simulink model "bldc_sim_abcFrame"  (R2024b)
settings: Solver=VariableStepAuto  StartTime=0.0  StopTime=2  RelTol=1e-3
values from neighbouring files (symbols this model uses):
  D_m = 1e-5    (= 1e-05)    [setup_motor_params.m]
  J = 12e-4    (= 0.0012)    [setup_motor_params.m]
  Ke = 0.1    [setup_motor_params.m]
  L_ss = 0.45e-3    (= 0.00045)    [setup_motor_params.m]
  P = 8    [setup_motor_params.m]
  phi_A_deg = 9.0 * 0    (= 0)    [setup_motor_params.m]
  phi_B_deg = -1.0 * 0    (= 0)    [setup_motor_params.m]
  phi_C_deg = 7.0* 0    (= 0)    [setup_motor_params.m]
  R_s = 0.15    [setup_motor_params.m]
  Ts_motor = 1e-6    (= 1e-06)    [setup_motor_params.m]
libraries: nesl_utility x12, ee_lib x6, fl_lib x5, embmathops x1, spsPWMGeneratorDCDCLib x1, simulink x1
settings Model: Creator=Aether  LastModifiedBy=Aether

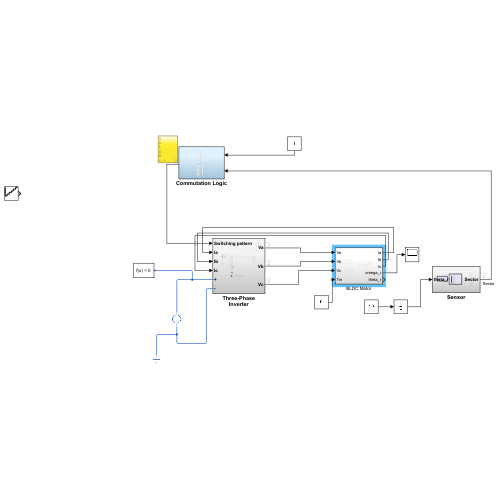
[thumbnail: Simulink's stored preview of the top-level diagram]
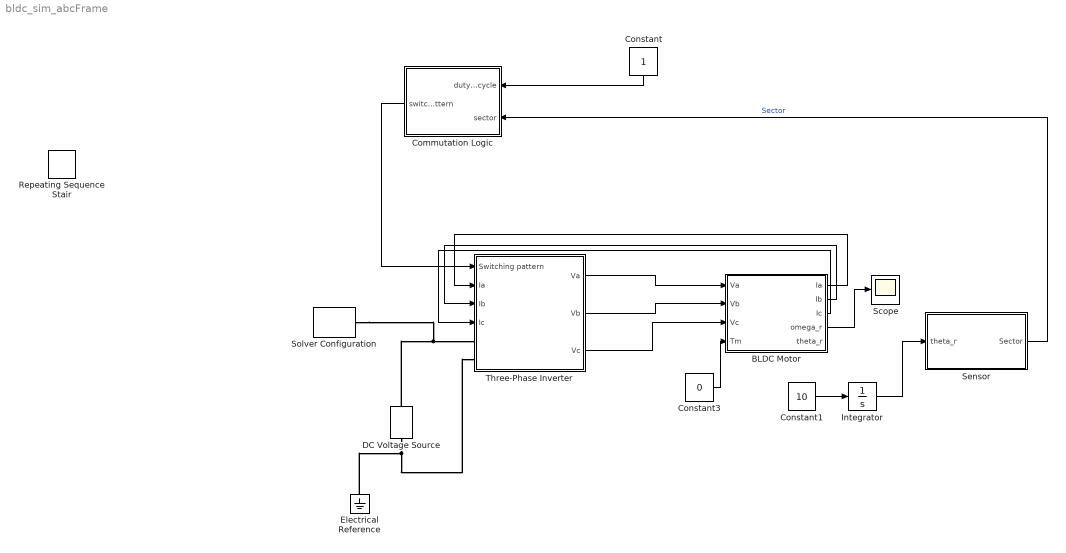
== system bldc_sim_abcFrame ==
  BLDC Motor : Subsystem
  Commutation Logic : Subsystem
  Constant : Constant
  Constant1 : Constant  Value=10
  Constant3 : Constant  Value=0
  DC Voltage Source : ee_lib/Additional Components/SPICE Sources/DC Voltage Source  DC=36 V
  Electrical Reference : fl_lib/Electrical/Electrical Elements/Electrical Reference
  Integrator : Integrator
  Repeating Sequence Stair : simulink/Sources/Repeating Sequence Stair  OutValues=[1 2 3 4 5 6]  tsamp=0.02  OutMin=[]  OutMax=[]  OutDataTypeStr=double  OutputDataTypeScalingMode=double  OutDataType=fixdt(0,8)  ConRadixGroup=Best Precision: Vector-wise  OutScaling=2^-12
  Scope : Scope
  Sensor : Subsystem
  Solver Configuration : nesl_utility/Solver Configuration  PhysicalDomain=network_engine_domain  SubClassName=solver  LeftPortType=input  RightPortType=generic  Tones=[]  Harmonics=[]  SimulateNoise=off  Profile=off  UseLocalSampling=off  EnableSwitchedLinearOptims=on  FrequencyDomain=off  UseCCode=off  RelTol=0.001  AbsTol=0.001  MinStep=1e-09  ToWorkspace=off  RevertToSquareIcSolve=off  NumHomotopyIterations=100  PhasorMode=off  PhasorModeNumHarmonics=1  ConsistencySolver=NEWTON_XTOL_AFTER_FTOL  IndexReductionMethod=DerivativeReplacement  DoDC=off  ResidualTolerance=1e-09  ConsistencyTolSource=GLOBAL  ConsistencyAbsTol=0.001  ConsistencyRelTol=0.001  ConsistencyTolFactor=0.001  UseLocalSolver=off  LocalSolverChoice=NE_BACKWARD_EULER_ADVANCER  ResolveIndetEquations=on  FunctionEvalNumThread=1  LocalSolverSampleTime=0.001  DoFixedCost=off  MaxNonlinIter=3  MaxModeIter=2  ComputeImpulses=off  ImpulseIterations=2  LinearAlgebra=auto  LinearAlgebraNumThread=0  EquationFormulation=NE_TIME_EF  DelaysMemoryBudget=1024  AutomaticFiltering=on  FilteringTimeConstant=0.001  PartitionStorageMethod=AS_NEEDED  PartitionMemoryBudget=1024  PartitionMethod=ROBUST  MultibodyUseLocalSolver=off  MultibodyLocalSolverChoice=ODE1  MultibodyLocalSolverSampleTime=0.001
  Three-Phase Inverter : Subsystem
  wires:
  Constant3/1 -> BLDC Motor/4(Tm)
  Constant/1 -> Commutation Logic/1(duty_cycle)
  BLDC Motor/1(Ia) -> Three-Phase Inverter/2(Ia)
  BLDC Motor/2(Ib) -> Three-Phase Inverter/3(Ib)
  BLDC Motor/3(Ic) -> Three-Phase Inverter/4(Ic)
  Three-Phase Inverter/1(Va) -> BLDC Motor/1(Va)
  Three-Phase Inverter/2(Vb) -> BLDC Motor/2(Vb)
  Three-Phase Inverter/3(Vc) -> BLDC Motor/3(Vc)
  BLDC Motor/4(omega_r) -> Scope/1
  Commutation Logic/1("  switching_pattern") -> Three-Phase Inverter/1(Switching pattern)
  Sensor/1(Sector) -> Commutation Logic/2(sector)  "Sector"
  Constant1/1 -> Integrator/1
  Integrator/1 -> Sensor/1(theta_r)
  connections:
  DC Voltage Source/LConn1 -- Solver Configuration/RConn1 -- Three-Phase Inverter/LConn1
  DC Voltage Source/RConn1 -- Electrical Reference/LConn1 -- Three-Phase Inverter/LConn2

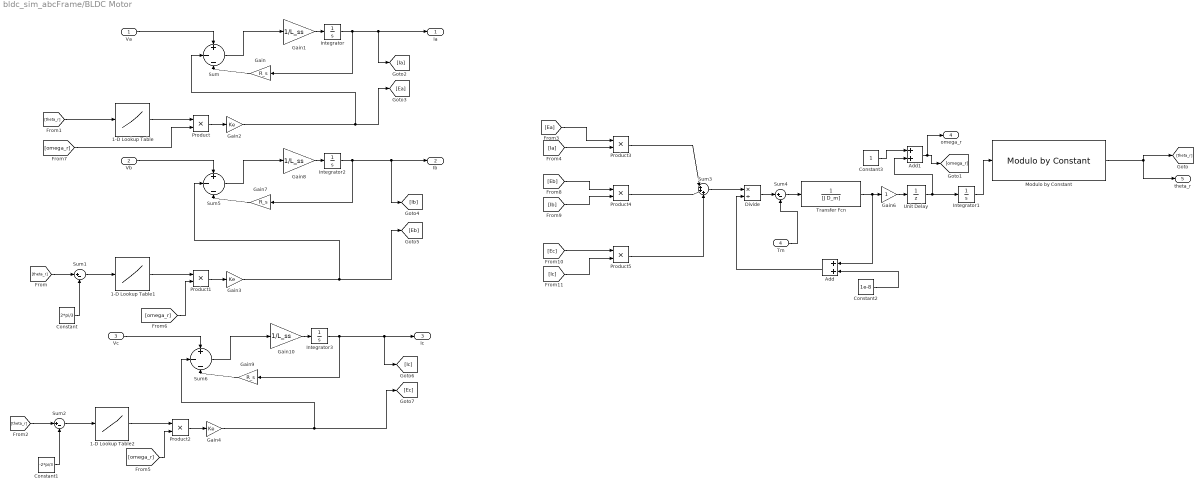
== system bldc_sim_abcFrame/BLDC Motor ==
  Va : Inport
  Vb : Inport  Port=2
  Vc : Inport  Port=3
  Tm : Inport  Port=4
  1-D Lookup Table : Lookup_n-D  NumberOfTableDimensions=1  BreakpointsForDimension1=[0, pi/3, 2*pi/3, pi, 4*pi/3, 5*pi/3, 2*pi]  Table=[0, 1, 1, 0, -1, -1, 0]  InternalRulePriority=Speed  RndMeth=Simplest
  1-D Lookup Table1 : Lookup_n-D  NumberOfTableDimensions=1  BreakpointsForDimension1=[0, pi/3, 2*pi/3, pi, 4*pi/3, 5*pi/3, 2*pi]  Table=[0, 1, 1, 0, -1, -1, 0]  InternalRulePriority=Speed  RndMeth=Simplest
  1-D Lookup Table2 : Lookup_n-D  NumberOfTableDimensions=1  BreakpointsForDimension1=[0, pi/3, 2*pi/3, pi, 4*pi/3, 5*pi/3, 2*pi]  Table=[0, 1, 1, 0, -1, -1, 0]  InternalRulePriority=Speed  RndMeth=Simplest
  Add : Sum
  Add1 : Sum
  Constant : Constant  Value=2*pi/3
  Constant1 : Constant  Value=-2*pi/3
  Constant2 : Constant  Value=1e-8
  Constant3 : Constant
  Divide : Product  Inputs=*/
  Gain : Gain  Gain=R_s
  Gain1 : Gain  Gain=1/L_ss
  Gain10 : Gain  Gain=1/L_ss
  Gain2 : Gain  Gain=Ke
  Gain3 : Gain  Gain=Ke
  Gain4 : Gain  Gain=Ke
  Gain6 : Gain
  Gain7 : Gain  Gain=R_s
  Gain8 : Gain  Gain=1/L_ss
  Gain9 : Gain  Gain=R_s
  Integrator : Integrator
  Integrator1 : Integrator  InitialCondition=0.1
  Integrator2 : Integrator
  Integrator3 : Integrator
  Modulo by Constant : embmathops/Modulo by Constant  Denominator=2*pi  SimulateUsing=Code generation
  Product{,1..5} (6 alike) : Product
  Sum : Sum  Inputs=+|-|-
  Sum1 : Sum  Inputs=|+-
  Sum2 : Sum  Inputs=|+-
  Sum3 : Sum  Inputs=|+++
  Sum4 : Sum  Inputs=|+-
  Sum5 : Sum  Inputs=+|-|-
  Sum6 : Sum  Inputs=+|-|-
  Transfer Fcn : TransferFcn  Denominator=[J D_m]
  Unit Delay : UnitDelay  SampleTime=-1  HasFrameUpgradeWarning=on
  Ia : Outport
  Ib : Outport  Port=2
  Ic : Outport  Port=3
  omega_r : Outport  Port=4
  theta_r : Outport  Port=5
  wires:
  Va/1 -> Sum/1
  Gain/1 -> Sum/3
  Sum/1 -> Gain1/1
  Gain1/1 -> Integrator/1
  Integrator/1 -> [Ia], Ia/1, Gain/1
  1-D Lookup Table/1 -> Product/1
  Product/1 -> Gain2/1
  Gain2/1 -> Sum/2, [Ea]
  Product1/1 -> Gain3/1
  1-D Lookup Table1/1 -> Product1/1
  Sum1/1 -> 1-D Lookup Table1/1
  Constant/1 -> Sum1/2
  Constant1/1 -> Sum2/2
  1-D Lookup Table2/1 -> Product2/1
  Product2/1 -> Gain4/1
  Sum2/1 -> 1-D Lookup Table2/1
  Product3/1 -> Sum3/1
  Product4/1 -> Sum3/2
  Product5/1 -> Sum3/3
  Sum3/1 -> Divide/1
  Divide/1 -> Sum4/1
  Tm/1 -> Sum4/2
  Sum4/1 -> Transfer Fcn/1
  Transfer Fcn/1 -> Gain6/1, Add/1
  Integrator1/1 -> Modulo by Constant/1
  Gain7/1 -> Sum5/3
  Gain8/1 -> Integrator2/1
  Sum5/1 -> Gain8/1
  Vb/1 -> Sum5/1
  Vc/1 -> Sum6/1
  Gain9/1 -> Sum6/3
  Gain10/1 -> Integrator3/1
  Sum6/1 -> Gain10/1
  Modulo by Constant/1 -> theta_r/1, [theta_r]
  [theta_r] -> Sum1/1
  [theta_r] -> Sum2/1
  [omega_r] -> Product2/2
  [omega_r] -> Product1/2
  [omega_r] -> Product/2
  [theta_r] -> 1-D Lookup Table/1
  Constant2/1 -> Add/2
  Add/1 -> Divide/2
  Gain3/1 -> Sum5/2, [Eb]
  Integrator2/1 -> [Ib], Ib/1, Gain7/1
  Integrator3/1 -> [Ic], Ic/1, Gain9/1
  Gain4/1 -> Sum6/2, [Ec]
  [Ea] -> Product3/1
  [Ia] -> Product3/2
  [Eb] -> Product4/1
  [Ib] -> Product4/2
  [Ec] -> Product5/1
  [Ic] -> Product5/2
  Gain6/1 -> Unit Delay/1
  Unit Delay/1 -> Integrator1/1, Add1/2
  Constant3/1 -> Add1/1
  Add1/1 -> omega_r/1, [omega_r]

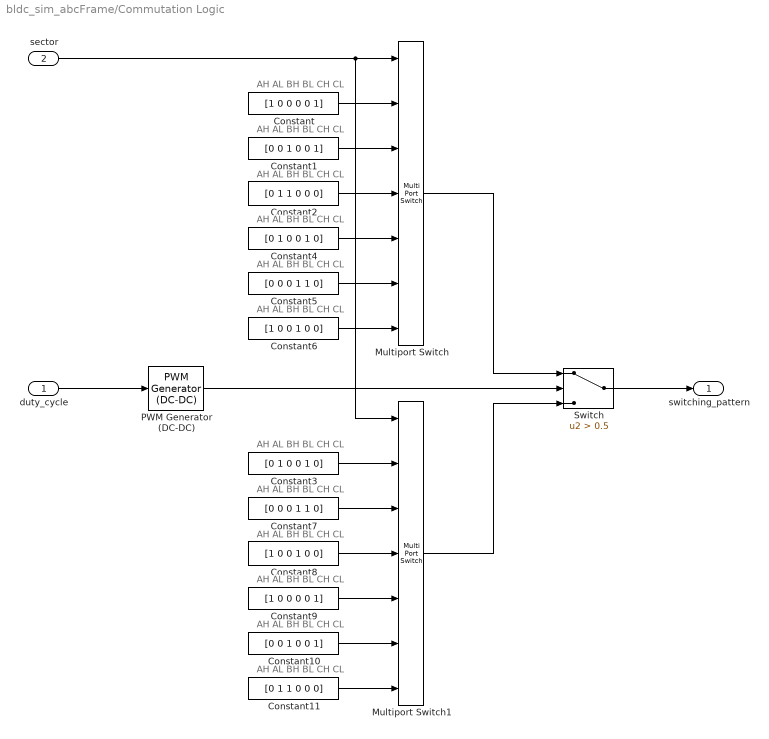
== system bldc_sim_abcFrame/Commutation Logic ==
  note: AH AL BH BL CH CL
  note: AH AL BH BL CH CL
  note: AH AL BH BL CH CL
  note: AH AL BH BL CH CL
  note: AH AL BH BL CH CL
  note: AH AL BH BL CH CL
  note: AH AL BH BL CH CL
  note: AH AL BH BL CH CL
  note: AH AL BH BL CH CL
  note: AH AL BH BL CH CL
  note: AH AL BH BL CH CL
  note: AH AL BH BL CH CL
  duty_cycle : Inport
  sector : Inport  Port=2
  Constant : Constant  Value=[1 0 0 0 0 1]
  Constant1 : Constant  Value=[0 0 1 0 0 1]
  Constant10 : Constant  Value=[0 0 1 0 0 1]
  Constant11 : Constant  Value=[0 1 1 0 0 0]
  Constant2 : Constant  Value=[0 1 1 0 0 0]
  Constant3 : Constant  Value=[0 1 0 0 1 0]
  Constant4 : Constant  Value=[0 1 0 0 1 0]
  Constant5 : Constant  Value=[0 0 0 1 1 0]
  Constant6 : Constant  Value=[1 0 0 1 0 0]
  Constant7 : Constant  Value=[0 0 0 1 1 0]
  Constant8 : Constant  Value=[1 0 0 1 0 0]
  Constant9 : Constant  Value=[1 0 0 0 0 1]
  Multiport Switch : MultiPortSwitch  Inputs=6  SaturateOnIntegerOverflow=off  InputSameDT=off
  Multiport Switch1 : MultiPortSwitch  Inputs=6  SaturateOnIntegerOverflow=off  InputSameDT=off
  PWM Generator (DC-DC) : spsPWMGeneratorDCDCLib/PWM Generator (DC-DC)  Fsw=1e7  Ts=Ts_motor
  Switch : Switch  Criteria=u2 > Threshold  Threshold=0.5  SaturateOnIntegerOverflow=off  InputSameDT=off
  "  switching_pattern" : Outport  VectorParamsAs1DForOutWhenUnconnected=off
  wires:
  Constant6/1 -> Multiport Switch/7
  Constant4/1 -> Multiport Switch/5
  sector/1 -> Multiport Switch1/1, Multiport Switch/1
  Constant1/1 -> Multiport Switch/3
  Constant2/1 -> Multiport Switch/4
  Constant5/1 -> Multiport Switch/6
  Constant/1 -> Multiport Switch/2
  Constant9/1 -> Multiport Switch1/5
  Constant11/1 -> Multiport Switch1/7
  Constant3/1 -> Multiport Switch1/2
  Constant7/1 -> Multiport Switch1/3
  Constant10/1 -> Multiport Switch1/6
  Constant8/1 -> Multiport Switch1/4
  PWM Generator (DC-DC)/1 -> Switch/2
  Switch/1 -> "  switching_pattern"/1
  Multiport Switch/1 -> Switch/1
  Multiport Switch1/1 -> Switch/3
  duty_cycle/1 -> PWM Generator (DC-DC)/1

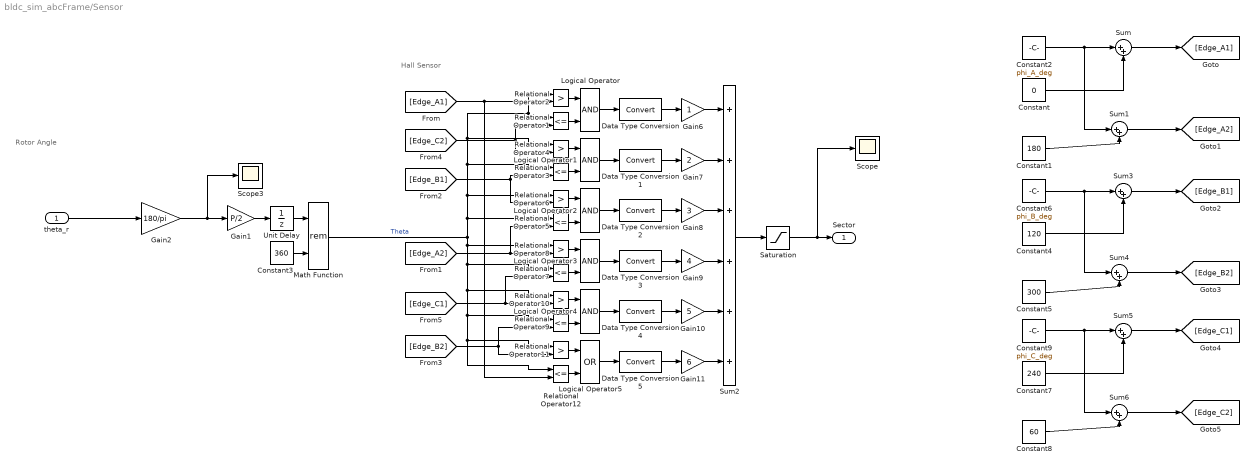
== system bldc_sim_abcFrame/Sensor ==
  note: Rotor Angle
  note: Hall Sensor
  theta_r : Inport
  Constant : Constant  Value=0
  Constant1 : Constant  Value=180
  Constant2 : Constant  Value=phi_A_deg
  Constant3 : Constant  Value=360
  Constant4 : Constant  Value=120
  Constant5 : Constant  Value=300
  Constant6 : Constant  Value=phi_B_deg
  Constant7 : Constant  Value=240
  Constant8 : Constant  Value=60
  Constant9 : Constant  Value=phi_C_deg
  Data Type Conversion{,1..5} (6 alike) : DataTypeConversion
  Gain1 : Gain  Gain=P/2
  Gain10 : Gain  Gain=5  SaturateOnIntegerOverflow=on  OutDataTypeStr=Inherit: Same as input  ParamDataTypeStr=Inherit: Same as input
  Gain11 : Gain  Gain=6  SaturateOnIntegerOverflow=on  OutDataTypeStr=Inherit: Same as input  ParamDataTypeStr=Inherit: Same as input
  Gain2 : Gain  Gain=180/pi
  Gain6 : Gain  SaturateOnIntegerOverflow=on  OutDataTypeStr=Inherit: Same as input  ParamDataTypeStr=Inherit: Same as input
  Gain7 : Gain  Gain=2  SaturateOnIntegerOverflow=on  OutDataTypeStr=Inherit: Same as input  ParamDataTypeStr=Inherit: Same as input
  Gain8 : Gain  Gain=3  SaturateOnIntegerOverflow=on  OutDataTypeStr=Inherit: Same as input  ParamDataTypeStr=Inherit: Same as input
  Gain9 : Gain  Gain=4  SaturateOnIntegerOverflow=on  OutDataTypeStr=Inherit: Same as input  ParamDataTypeStr=Inherit: Same as input
  Logical Operator{,1..4} (5 alike) : Logic
  Logical Operator5 : Logic  Operator=OR
  Math Function : Math  Operator=rem  SignedPower=on
  Relational Operator{1,3,5,7,9,12} (6 alike) : RelationalOperator  Operator=<=
  Relational Operator{2,4,6,8,10..11} (6 alike) : RelationalOperator  Operator=>
  Saturation : Saturate  UpperLimit=6  LowerLimit=1
  Scope : Scope
  Scope3 : Scope
  Sum{,1,3..6} (6 alike) : Sum  Inputs=|++
  Sum2 : Sum  Inputs=++++++  InputSameDT=on  SaturateOnIntegerOverflow=on  OutDataTypeStr=Inherit: Same as first input
  Unit Delay : UnitDelay  SampleTime=Ts_motor  HasFrameUpgradeWarning=on
  Sector : Outport
  wires:
  Saturation/1 -> Scope/1, Sector/1
  Math Function/1 -> Relational Operator2/1, Relational Operator1/1, Relational Operator4/1, Relational Operator3/1, Relational Operator6/1, Relational Operator5/1, Relational Operator12/1, Relational Operator11/1, Relational Operator9/1, Relational Operator10/1, Relational Operator7/1, Relational Operator8/1  "Theta"
  Data Type Conversion5/1 -> Gain11/1
  Data Type Conversion4/1 -> Gain10/1
  Data Type Conversion3/1 -> Gain9/1
  Data Type Conversion2/1 -> Gain8/1
  Data Type Conversion1/1 -> Gain7/1
  Data Type Conversion/1 -> Gain6/1
  Relational Operator2/1 -> Logical Operator/1
  Relational Operator1/1 -> Logical Operator/2
  Logical Operator/1 -> Data Type Conversion/1
  [Edge_A1] -> Relational Operator12/2, Relational Operator2/2
  Relational Operator4/1 -> Logical Operator1/1
  Relational Operator3/1 -> Logical Operator1/2
  Logical Operator1/1 -> Data Type Conversion1/1
  [Edge_C2] -> Relational Operator1/2, Relational Operator4/2
  Relational Operator6/1 -> Logical Operator2/1
  Relational Operator5/1 -> Logical Operator2/2
  Logical Operator2/1 -> Data Type Conversion2/1
  Relational Operator8/1 -> Logical Operator3/1
  Relational Operator7/1 -> Logical Operator3/2
  Logical Operator3/1 -> Data Type Conversion3/1
  Relational Operator10/1 -> Logical Operator4/1
  Relational Operator9/1 -> Logical Operator4/2
  Logical Operator4/1 -> Data Type Conversion4/1
  Relational Operator11/1 -> Logical Operator5/1
  Relational Operator12/1 -> Logical Operator5/2
  Logical Operator5/1 -> Data Type Conversion5/1
  Gain6/1 -> Sum2/1
  Gain7/1 -> Sum2/2
  Gain8/1 -> Sum2/3
  Gain9/1 -> Sum2/4
  Gain10/1 -> Sum2/5
  Gain11/1 -> Sum2/6
  Sum2/1 -> Saturation/1
  Gain2/1 -> Scope3/1, Gain1/1
  Constant3/1 -> Math Function/2
  Gain1/1 -> Unit Delay/1
  Unit Delay/1 -> Math Function/1
  Constant/1 -> Sum/2
  Constant2/1 -> Sum1/1, Sum/1
  Constant1/1 -> Sum1/2
  Sum/1 -> [Edge_A1]
  Sum1/1 -> [Edge_A2]
  Constant6/1 -> Sum4/1, Sum3/1
  Constant5/1 -> Sum4/2
  Constant4/1 -> Sum3/2
  Sum3/1 -> [Edge_B1]
  Sum4/1 -> [Edge_B2]
  Constant9/1 -> Sum6/1, Sum5/1
  Constant8/1 -> Sum6/2
  Constant7/1 -> Sum5/2
  Sum5/1 -> [Edge_C1]
  Sum6/1 -> [Edge_C2]
  [Edge_B1] -> Relational Operator3/2, Relational Operator6/2
  [Edge_A2] -> Relational Operator5/2, Relational Operator8/2
  [Edge_C1] -> Relational Operator7/2, Relational Operator10/2
  [Edge_B2] -> Relational Operator11/2, Relational Operator9/2
  theta_r/1 -> Gain2/1

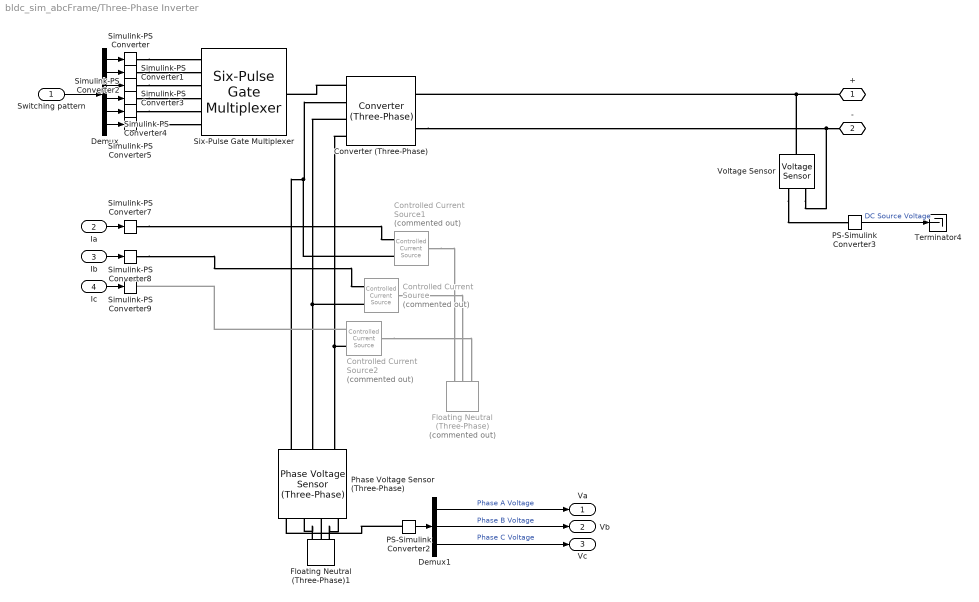
== system bldc_sim_abcFrame/Three-Phase Inverter ==
  Switching pattern : Inport
  Ia : Inport  Port=2
  Ib : Inport  Port=3
  Ic : Inport  Port=4
  Controlled Current Source : fl_lib/Electrical/Electrical Sources/Controlled Current Source  Commented=on
  Controlled Current Source1 : fl_lib/Electrical/Electrical Sources/Controlled Current Source  Commented=on
  Controlled Current Source2 : fl_lib/Electrical/Electrical Sources/Controlled Current Source  Commented=on
  Converter (Three-Phase) : ee_lib/Semiconductors & Converters/Converters/Converter (Three-Phase)  port_option=ee.enum.threePhasePort.expanded  fidelity_option=ee.enum.converters.fidelity.detailed  device_type=ee.enum.converters.switchingdevice.ideal  showThermalPort=false  K=0  Vth=0.5 V  Vgt=1 V  Vgt_off=-1 V  Ih=1 A  Vf=0.8 V  Ron=0.001 Ohm  Rds=0.001 Ohm  Goff=0.001 1/Ohm  Eon_scalar=22.86e-3 J  Eoff_scalar=17.14e-3 J  Eoff_natural_commutation=10e-3 J  Voff=300 V  Iout_scalar=600 A  onCurrentMeasDelay=0 s  useCurrentFromPreviousCycle=false  useVoltageFromPreviousCycle=false  diode_param=ee.enum.converters.protectiondiode.nodynamics  diode_Vf=0.8 V  diode_Ron=0.001 Ohm  diode_Goff=1e-5 1/Ohm  diode_C=50 nF  diode_iRM=-235 A  diode_iF=300 A  diode_idot=-50 A/us  diode_trr_param=ee.enum.converters.diodetrr.trr_factor  diode_trr_factor=3  diode_trr=15 us  diode_Qrr=1500 s*uA  diode_rec_loss_model=ee.enum.diode.reverseRecoveryModel.fixed  diode_ErecVal=0 J  diode_scaleWithIandV=false  diode_ErecMat=zeros(2, 3) J  diode_TjrecVec=[298.15, 398.15] K  diode_IfrecVec=[.1, 1, 10] A  diode_IrecVal=10 A  diode_VrecVal=10 V  diode_tFilter=1 / 1000 / 100 s  thermal_network_parameterization=ee.enum.thermalNetworkTopology.external  Rth=[.08, .5] K/W  Rth_Cauer=[.08, .1, .5] K/W  Rth_Foster=[.08, .14, .22, .16] K/W  thermal_mass_parameterization=ee.enum.thermalNetwork.timeconstant  thermal_mass=[.01, .5] J/K  thermal_mass_Cauer=[.01, .1, .5] J/K  thermal_mass_Foster=[.001, .005, .05, .5] J/K  thermal_time_constant=[.001, .2] s  thermal_time_constant_Cauer=[.001, .1, .2] s  thermal_time_constant_Foster=[7e-05, .0007, .01, .08] s  thermal_mass_initial_temperatures=[25, 25] degC  thermal_mass_initial_temperatures_Cauer=[25, 25, 25] degC  junction_thermal_mass=0.01 J/K  Tvec_initial_Foster=[25, 25, 25, 25] degC  snubber_type=ee.enum.converters.snubber.exclude  Cs=1e-7 F  Rs=0.1 Ohm  Vce_loss=[0, 150, 300] V
      settings: InternalSimscapePortConfiguration="{\"Bottom\":[],\"Left\":[{\"id\":\"G\",\"label\":\"G\",\"type\":\"foundation.electrical.twelve_phase\"},{\"id\":\"a\",\"label\":\"a\",\"type\":\"foundation.electrical.electrical\"},{\"id\":\"b\",\"label\":\"b\",\"type\":\"foundation.electrical.electrical\"},{\"id\":\"c\",\"label\":\"c\",\"type\":\"foundation.electrical.electrical\"}],\"Right\":[{\"id\":\"p\",\"label\":\"+\",\"type\":\"foundation.electrical.electrical\"},{\"id\":\"n\",\"label\":\"-\",\"type\":\"foundation.electrical.electrical\"}],\"Top\":[]}"
  Demux : Demux  Outputs=6
  Demux1 : Demux  Outputs=3
  Floating Neutral (Three-Phase) : ee_lib/Connectors & References/Floating Neutral (Three-Phase)  Commented=on  G_parasitic=1e-12 1/Ohm
      settings: InternalSimscapePortConfiguration="{\"Bottom\":[],\"Left\":[{\"id\":\"a\",\"label\":\"a\",\"type\":\"foundation.electrical.electrical\"},{\"id\":\"b\",\"label\":\"b\",\"type\":\"foundation.electrical.electrical\"},{\"id\":\"c\",\"label\":\"c\",\"type\":\"foundation.electrical.electrical\"}],\"Right\":[],\"Top\":[]}"
  Floating Neutral (Three-Phase)1 : ee_lib/Connectors & References/Floating Neutral (Three-Phase)  G_parasitic=1e-12 1/Ohm
      settings: InternalSimscapePortConfiguration="{\"Bottom\":[],\"Left\":[{\"id\":\"a\",\"label\":\"a\",\"type\":\"foundation.electrical.electrical\"},{\"id\":\"b\",\"label\":\"b\",\"type\":\"foundation.electrical.electrical\"},{\"id\":\"c\",\"label\":\"c\",\"type\":\"foundation.electrical.electrical\"}],\"Right\":[],\"Top\":[]}"
  PS-Simulink Converter2 : nesl_utility/PS-Simulink Converter  PhysicalDomain=network_engine_domain  SubClassName=ps_output  LeftPortType=input  RightPortType=output  PseudoPeriodic=off  Frequencies=[]  VectorFormat=1-D array  Unit=inherit  AffineConversion=off
  PS-Simulink Converter3 : nesl_utility/PS-Simulink Converter  PhysicalDomain=network_engine_domain  SubClassName=ps_output  LeftPortType=input  RightPortType=output  PseudoPeriodic=off  Frequencies=[]  VectorFormat=1-D array  Unit=inherit  AffineConversion=off
  Phase Voltage Sensor (Three-Phase) : ee_lib/Sensors & Transducers/Phase Voltage Sensor (Three-Phase)
      settings: InternalSimscapePortConfiguration="{\"Bottom\":[],\"Left\":[{\"id\":\"a1\",\"label\":\"a1\",\"type\":\"foundation.electrical.electrical\"},{\"id\":\"b1\",\"label\":\"b1\",\"type\":\"foundation.electrical.electrical\"},{\"id\":\"c1\",\"label\":\"c1\",\"type\":\"foundation.electrical.electrical\"}],\"Right\":[{\"id\":\"V_output\",\"label\":\"V\",\"type\":\"output\"},{\"id\":\"a2\",\"label\":\"a2\",\"type\":\"foundation.electrical.electrical\"},{\"id\":\"b2\",\"label\":\"b2\",\"type\":\"foundation.electrical.electrical\"},{\"id\":\"c2\",\"label\":\"c2\",\"type\":\"foundation.electrical.electrical\"}],\"Top\":[]}"
  Simulink-PS Converter{,1..5,7..9} (9 alike) : nesl_utility/Simulink-PS Converter  PhysicalDomain=network_engine_domain  SubClassName=ps_input  LeftPortType=input  RightPortType=output  PseudoPeriodic=off  Frequencies=[]  NoiseDistribution=none  NoiseParameters=[]  Unit=1  AffineConversion=off  FilteringAndDerivatives=provide  SimscapeFilterOrder=1  InputFilterTimeConstant=0.001  UdotUserProvided=0
  Six-Pulse Gate Multiplexer : ee_lib/Semiconductors & Converters/Converters/Six-Pulse Gate Multiplexer  port_option=ee.enum.controlport.ps
  Terminator4 : Terminator
  Voltage Sensor : fl_lib/Electrical/Electrical Sensors/Voltage Sensor
  + : PMIOPort  Side=Left
  - : PMIOPort  Port=2  Side=Left
  Va : Outport
  Vb : Outport  Port=2
  Vc : Outport  Port=3
  wires:
  Switching pattern/1 -> Demux/1
  Demux/1 -> Simulink-PS Converter/1
  Demux/2 -> Simulink-PS Converter1/1
  Demux/3 -> Simulink-PS Converter2/1
  Demux/4 -> Simulink-PS Converter3/1
  Demux/5 -> Simulink-PS Converter4/1
  Demux/6 -> Simulink-PS Converter5/1
  PS-Simulink Converter2/1 -> Demux1/1
  Demux1/1 -> Va/1  "Phase A Voltage"
  Demux1/2 -> Vb/1  "Phase B Voltage"
  Demux1/3 -> Vc/1  "Phase C Voltage"
  PS-Simulink Converter3/1 -> Terminator4/1  "DC Source Voltage"
  Ia/1 -> Simulink-PS Converter7/1
  Ib/1 -> Simulink-PS Converter8/1
  Ic/1 -> Simulink-PS Converter9/1
  connections:
  Simulink-PS Converter/RConn1 -- Six-Pulse Gate Multiplexer/LConn1
  Simulink-PS Converter1/RConn1 -- Six-Pulse Gate Multiplexer/LConn2
  Simulink-PS Converter2/RConn1 -- Six-Pulse Gate Multiplexer/LConn3
  Simulink-PS Converter3/RConn1 -- Six-Pulse Gate Multiplexer/LConn4
  Simulink-PS Converter4/RConn1 -- Six-Pulse Gate Multiplexer/LConn5
  Simulink-PS Converter5/RConn1 -- Six-Pulse Gate Multiplexer/LConn6
  Converter (Three-Phase)/LConn1 -- Six-Pulse Gate Multiplexer/RConn1
  +/RConn1 -- Voltage Sensor/LConn1 -- Converter (Three-Phase)/RConn1
  Converter (Three-Phase)/RConn2 -- Voltage Sensor/RConn2 -- -/RConn1
  Phase Voltage Sensor (Three-Phase)/LConn1 -- Controlled Current Source1/RConn2 -- Converter (Three-Phase)/LConn2
  PS-Simulink Converter2/LConn1 -- Phase Voltage Sensor (Three-Phase)/RConn1
  Voltage Sensor/RConn1 -- PS-Simulink Converter3/LConn1
  Converter (Three-Phase)/LConn3 -- Controlled Current Source/RConn2 -- Phase Voltage Sensor (Three-Phase)/LConn2
  Converter (Three-Phase)/LConn4 -- Controlled Current Source2/RConn2 -- Phase Voltage Sensor (Three-Phase)/LConn3
  Simulink-PS Converter7/RConn1 -- Controlled Current Source1/RConn1
  Simulink-PS Converter8/RConn1 -- Controlled Current Source/RConn1
  Controlled Current Source2/RConn1 -- Simulink-PS Converter9/RConn1
  Controlled Current Source/LConn1 -- Floating Neutral (Three-Phase)/LConn2
  Controlled Current Source1/LConn1 -- Floating Neutral (Three-Phase)/LConn1
  Controlled Current Source2/LConn1 -- Floating Neutral (Three-Phase)/LConn3
  Floating Neutral (Three-Phase)1/LConn1 -- Phase Voltage Sensor (Three-Phase)/RConn2
  Floating Neutral (Three-Phase)1/LConn2 -- Phase Voltage Sensor (Three-Phase)/RConn3
  Floating Neutral (Three-Phase)1/LConn3 -- Phase Voltage Sensor (Three-Phase)/RConn4
